simulink model "suspension"  (R2019a)
settings: Solver=ode15s  StartTime=0.0  StopTime=60  MaxStep=0.01  RelTol=1e-3  EnableMultiTasking=on
model workspace (MATLAB code in the model file):
  | dgrey = [0.3 0.3 0.3];
  | lgrey = [0.6 0.6 0.6];
  | orange = [255 140 0]/255;
  | blue = [0.0 0.6 0.8];
  | brown = [0.3 0.2 0.0];
  | lbrown = [167 108 52]/255;
  | yellow = [0.9 0.7 0.2];
  | red = [1.0 0.2 0.2];
  | black = [0 0 0];
  | 
  | rho_alum = 2700;
values from neighbouring files (symbols this model uses):
  back_frame_rad = intocm(0.25)    [loading.m]
  back_frame_thick_frame = intocm(0.25)    [loading.m]
  brake_disk_rad = intocm(3)    [loading.m]
  brake_disk_thick = intocm(0.25)    [loading.m]
  front_frame_rad = intocm(0.25)    [loading.m]
  front_frame_thick_frame = intocm(0.25)    [loading.m]
  hub_radius = intocm(2)    [loading.m]
  lower_left_link_len = intocm(link_upper)    [loading.m]
  lower_right_link_len = intocm(link_upper)    [loading.m]
  max_angle = 35    [loading.m]
  num_spokes = 4    [loading.m]
  outer_radius_spokes = intocm(5)    [loading.m]
  shaft_len = intocm(8)    [loading.m]
  shaft_rad = intocm(1.5)    [loading.m]
  steer_arm_chamfer = 0.25    [loading.m]
  steer_arm_height_forked = 13    [loading.m]
  steer_arm_len = 20    [loading.m]
  steer_arm_len_forked = 4    [loading.m]
  steer_arm_offset_forked = 3    [loading.m]
  steer_arm_pin_rad = 0.25    [loading.m]
  steer_arm_thick = 1    [loading.m]
  steer_arm_width = 2    [loading.m]
  steering_ball_rad = 1    [loading.m]
  steering_pin_height = 3    [loading.m]
  steering_pin_rad = 0.5    [loading.m]
  thickness_spokes = intocm(1)    [loading.m]
  tire_chamfer = 1    [loading.m]
  tire_density = 1000    [loading.m]
  tire_radius = intocm(9)    [loading.m]
  tire_width = intocm(7.5)    [loading.m]
  Ts = 60    [loading.m]
  upper_left_link_len = intocm(link_upper)    [loading.m]
  upper_right_link_len = intocm(link_upper)    [loading.m]
  upright_bearing_housing = 6    [loading.m]
  upright_chamfer = 0.3    [loading.m]
  upright_heigh_wheel = 8    [loading.m]
  upright_height = 43    [loading.m]
  upright_hub_thick = 2.5    [loading.m]
  upright_len = 8    [loading.m]
  upright_shaft_rad = 2.5    [loading.m]
  upright_thickness = 1    [loading.m]
  upright_trans_rad_to_wheel = 2    [loading.m]
  upright_width_wishbone = 10    [loading.m]
  width_hub = intocm(4.5)    [loading.m]
undefined symbols (not defined in the file or in its folder): sm_dwb_roadgen, X, Y, Z
libraries: sm_lib x75, sm_double_wishbone_suspension_lib x23, nesl_utility x18, simulink x3
(part 1 of 4)
Description:
  | Double Wishbone Suspension
  | 
  | This example illustrates a double wishbone front wheel automotive suspension. The suspension is
  | mounted on two platforms that can independently move up and down to simulate a road profile on
  | each wheel. For a given pair of road profiles, the resultant roll and bounce of the chassis can be
  | studied and the suspension parameters tuned for optimal performance. The inputs to the two
  | platforms are the road profile and its derivative. The platforms have a PD controller that controls
  | the vertical position of the platform to mimic the input road profile. See "Road Profiles Generator"
  | block dialog for details on the test road profiles.
  | 
  | Copyright 2008-2019 The MathWorks, Inc.
settings Model: Creator=MathWorks  LastModifiedBy=nicwiggins
settings DataIOCC: LimitDataPoints=on  SaveFormat=Array  SaveOutput=off  SaveTime=off  ReturnWorkspaceOutputs=off
settings OptimizationCC: ExpressionDepthLimit=2147483647  LifeSpan=inf
settings DebuggingCC: UnderspecifiedInitializationDetection=Classic  MergeDetectMultiDrivingBlocksExec=none  AllowSymbolicDim=off  StateNameClashWarn=warning  SFUnexpectedBacktrackingDiag=warning  SFNoUnconditionalDefaultTransitionDiag=warning  SFExecutionAtInitializationDiag=none  ArithmeticOperatorsInVariantConditions=warning
settings HardwareCC: ProdBitPerPointer=32  ProdBitPerSizeT=32  ProdBitPerPtrDiffT=32  ProdLargestAtomicFloat=None  ProdIntDivRoundTo=Undefined  ProdEndianess=Unspecified  ProdWordSize=32  ProdHWDeviceType=32-bit Generic
settings ModelReferenceCC: PropagateSignalLabelsOutOfModel=off
settings SFSimCC: SimUseLocalCustomCode=off  SimBuildMode=sf_make
settings RTWCC: RTWUseLocalCustomCode=off
settings CodeAppCC: StateflowObjectComments=on
settings GRTTargetCC: TargetLangStandard=C89/C90 (ANSI)  GeneratePreprocessorConditionals=Disable all
settings ConfigComp: CovMetricSettings=dw  CovHtmlReporting=on  CovSaveCumulativeToWorkspaceVar=on  CovSaveSingleToWorkspaceVar=on  CovExternalEMLEnable=off  CovSFcnEnable=off
settings SimscapeCC: SimscapeNormalizeSystem=off
settings ConfigurationSet: Description=SimMechanics 2G
settings DiagnosticsConfigSet: SimMechanicsUnconnectedFramePorts=none
settings ExplorerConfigSet: InternalSimMechanicsExplorerSettings="<ExplorerConfiguration><canonicalview>default</canonicalview><AnimationSetting><BasePlaybackSpeed>1.0</BasePlaybackSpeed><PlaybackSpeedFactor>1.0</PlaybackSpeedFactor></AnimationSetting><TilePanel><TileInfo><Tiles Columns=\"1\" Count=\"1\" Rows=\"1\"><Column Left=\"2\" Weight=\"1\"/><Column Left=\"827\"/><Row Top=\"2\" Weight=\"1\"/><Row Top=\"666\"/><Tile Height=\"1\" Width=\"1\" X=\"0\" Y=\"0\"/></Tiles></TileInfo><SceneInfo><SceneViewer><BGColor><R>0.60000002384185791</R><G>0.60000002384185791</G><B>0.60000002384185791</B></BGColor><Camera><Position><X>0</X><Y>-4.48140033882927202</Y><Z>0.554502487182617188</Z></Position><Center><X>0</X><Y>-0.245328903198242188</Y><Z>0.554502487182617188</Z></Center><Up><X>0</X><Y>-0</Y><Z>1</Z></Up><Left>-1.15500002503395094</Left><Right>1.15500002503395094</Right><Bottom>-0.792227599024772688</Bottom><Top>0.792227599024772688</Top></Camera></SceneViewer></SceneInfo></TilePanel></ExplorerConfiguration>"

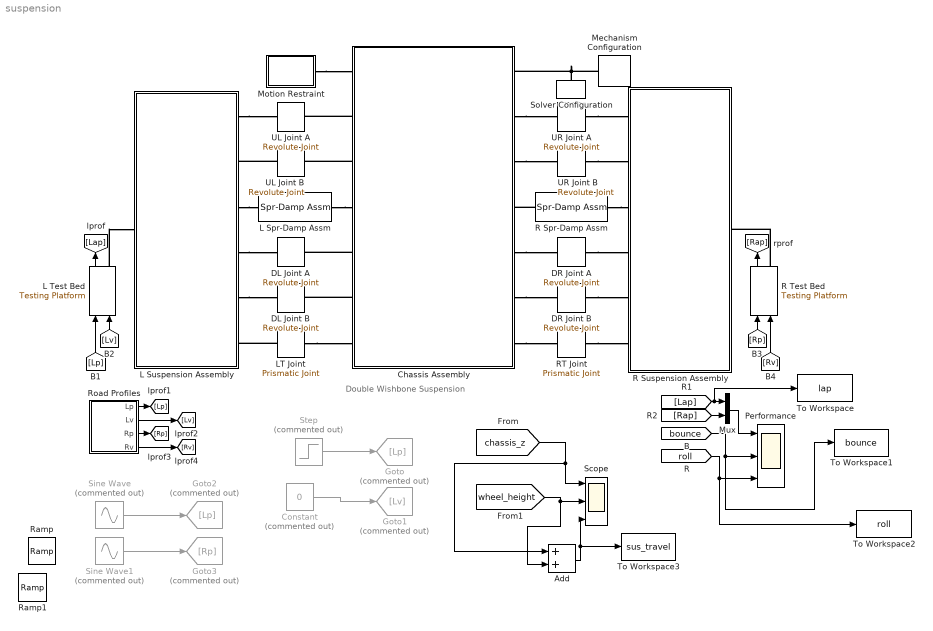
== system suspension ==
  note: Double Wishbone Suspension
  Add : Sum
  Chassis Assembly : Subsystem
      mask Display:
      | image(imread('sm_dwishbone_frameassm.png'));
      | port_label('LConn',1,'BC');
      | port_label('LConn',2,'ULA');
      | port_label('LConn',3,'ULB');
      | port_label('LConn',4,'ULC');
      | port_label('LConn',5,'DLA');
      | port_label('LConn',6,'DLB');
      | port_label('LConn',7,'LT');
      | port_label('RConn',1,'FC');
      | port_label('RConn',2,'URA');
      | port_label('RConn',3,'URB');
      | port_label('RConn',4,'URC');
      | port_label('RConn',5,'DRA');
      | port_label('RConn',6,'DRB');
      | port_label('RConn',7,'RT');
  Constant : Constant  Commented=on  Value=0
  DL Joint A : sm_lib/Joints/Revolute Joint  SenseConstraintForce=off  SenseConstraintForceX=off  SenseConstraintForceY=off  SenseConstraintForceZ=off  SenseConstraintTorque=off  SenseConstraintTorqueX=off  SenseConstraintTorqueY=off  SenseConstraintTorqueZ=off  SenseTotalForce=off  SenseTotalForceX=off  SenseTotalForceY=off  SenseTotalForceZ=off  SenseTotalTorque=off  SenseTotalTorqueX=off  SenseTotalTorqueY=off  SenseTotalTorqueZ=off  CompositeWrenchDir=FollowerOnBase  CompositeWrenchFrame=BaseFrame  EquilibriumPosition=0  EquilibriumPositionUnits=deg  SpringStiffness=0  SpringStiffnessUnits=N*m/deg  DampingCoefficient=0  DampingCoefficientUnits=N*m/(deg/s)  TorqueActuationMode=NoTorque  MotionActuationMode=ComputedMotion  SensePosition=off  SenseVelocity=off  SenseAcceleration=off  SenseTorqueForce=off  SenseLowerLimitTorqueForce=off  SenseUpperLimitTorqueForce=off  LowerLimitSpecify=off  LowerLimitBound=-90  LowerLimitBoundUnits=deg  LowerLimitStiffness=1e4  LowerLimitStiffnessUnits=N*m/deg  LowerLimitDamping=10  LowerLimitDampingUnits=N*m/(deg/s)  LowerLimitTransitionRegionWidth=0.1  LowerLimitTransitionRegionWidthUnits=deg  UpperLimitSpecify=off  UpperLimitBound=90  UpperLimitBoundUnits=deg  UpperLimitStiffness=1e4  UpperLimitStiffnessUnits=N*m/deg  UpperLimitDamping=10  UpperLimitDampingUnits=N*m/(deg/s)  UpperLimitTransitionRegionWidth=0.1  UpperLimitTransitionRegionWidthUnits=deg  PositionTargetSpecify=on  PositionTargetPriority=High  PositionTargetValue=0  PositionTargetValueUnits=deg  VelocityTargetSpecify=off  VelocityTargetPriority=High  VelocityTargetValue=0  VelocityTargetValueUnits=deg/s
  DL Joint B : sm_lib/Joints/Revolute Joint  SenseConstraintForce=off  SenseConstraintForceX=off  SenseConstraintForceY=off  SenseConstraintForceZ=off  SenseConstraintTorque=off  SenseConstraintTorqueX=off  SenseConstraintTorqueY=off  SenseConstraintTorqueZ=off  SenseTotalForce=off  SenseTotalForceX=off  SenseTotalForceY=off  SenseTotalForceZ=off  SenseTotalTorque=off  SenseTotalTorqueX=off  SenseTotalTorqueY=off  SenseTotalTorqueZ=off  CompositeWrenchDir=FollowerOnBase  CompositeWrenchFrame=BaseFrame  EquilibriumPosition=0  EquilibriumPositionUnits=deg  SpringStiffness=0  SpringStiffnessUnits=N*m/deg  DampingCoefficient=0  DampingCoefficientUnits=N*m/(deg/s)  TorqueActuationMode=NoTorque  MotionActuationMode=ComputedMotion  SensePosition=off  SenseVelocity=off  SenseAcceleration=off  SenseTorqueForce=off  SenseLowerLimitTorqueForce=off  SenseUpperLimitTorqueForce=off  LowerLimitSpecify=off  LowerLimitBound=-90  LowerLimitBoundUnits=deg  LowerLimitStiffness=1e4  LowerLimitStiffnessUnits=N*m/deg  LowerLimitDamping=10  LowerLimitDampingUnits=N*m/(deg/s)  LowerLimitTransitionRegionWidth=0.1  LowerLimitTransitionRegionWidthUnits=deg  UpperLimitSpecify=off  UpperLimitBound=90  UpperLimitBoundUnits=deg  UpperLimitStiffness=1e4  UpperLimitStiffnessUnits=N*m/deg  UpperLimitDamping=10  UpperLimitDampingUnits=N*m/(deg/s)  UpperLimitTransitionRegionWidth=0.1  UpperLimitTransitionRegionWidthUnits=deg  PositionTargetSpecify=off  PositionTargetPriority=High  PositionTargetValue=90  PositionTargetValueUnits=deg  VelocityTargetSpecify=off  VelocityTargetPriority=High  VelocityTargetValue=0  VelocityTargetValueUnits=deg/s
  DR Joint A : sm_lib/Joints/Revolute Joint  SenseConstraintForce=off  SenseConstraintForceX=off  SenseConstraintForceY=off  SenseConstraintForceZ=off  SenseConstraintTorque=off  SenseConstraintTorqueX=off  SenseConstraintTorqueY=off  SenseConstraintTorqueZ=off  SenseTotalForce=off  SenseTotalForceX=off  SenseTotalForceY=off  SenseTotalForceZ=off  SenseTotalTorque=off  SenseTotalTorqueX=off  SenseTotalTorqueY=off  SenseTotalTorqueZ=off  CompositeWrenchDir=FollowerOnBase  CompositeWrenchFrame=BaseFrame  EquilibriumPosition=0  EquilibriumPositionUnits=deg  SpringStiffness=0  SpringStiffnessUnits=N*m/deg  DampingCoefficient=0  DampingCoefficientUnits=N*m/(deg/s)  TorqueActuationMode=NoTorque  MotionActuationMode=ComputedMotion  SensePosition=off  SenseVelocity=off  SenseAcceleration=off  SenseTorqueForce=off  SenseLowerLimitTorqueForce=off  SenseUpperLimitTorqueForce=off  LowerLimitSpecify=off  LowerLimitBound=-90  LowerLimitBoundUnits=deg  LowerLimitStiffness=1e4  LowerLimitStiffnessUnits=N*m/deg  LowerLimitDamping=10  LowerLimitDampingUnits=N*m/(deg/s)  LowerLimitTransitionRegionWidth=0.1  LowerLimitTransitionRegionWidthUnits=deg  UpperLimitSpecify=off  UpperLimitBound=90  UpperLimitBoundUnits=deg  UpperLimitStiffness=1e4  UpperLimitStiffnessUnits=N*m/deg  UpperLimitDamping=10  UpperLimitDampingUnits=N*m/(deg/s)  UpperLimitTransitionRegionWidth=0.1  UpperLimitTransitionRegionWidthUnits=deg  PositionTargetSpecify=on  PositionTargetPriority=High  PositionTargetValue=0  PositionTargetValueUnits=deg  VelocityTargetSpecify=off  VelocityTargetPriority=High  VelocityTargetValue=0  VelocityTargetValueUnits=deg/s
  DR Joint B : sm_lib/Joints/Revolute Joint  SenseConstraintForce=off  SenseConstraintForceX=off  SenseConstraintForceY=off  SenseConstraintForceZ=off  SenseConstraintTorque=off  SenseConstraintTorqueX=off  SenseConstraintTorqueY=off  SenseConstraintTorqueZ=off  SenseTotalForce=off  SenseTotalForceX=off  SenseTotalForceY=off  SenseTotalForceZ=off  SenseTotalTorque=off  SenseTotalTorqueX=off  SenseTotalTorqueY=off  SenseTotalTorqueZ=off  CompositeWrenchDir=FollowerOnBase  CompositeWrenchFrame=BaseFrame  EquilibriumPosition=0  EquilibriumPositionUnits=deg  SpringStiffness=0  SpringStiffnessUnits=N*m/deg  DampingCoefficient=0  DampingCoefficientUnits=N*m/(deg/s)  TorqueActuationMode=NoTorque  MotionActuationMode=ComputedMotion  SensePosition=off  SenseVelocity=off  SenseAcceleration=off  SenseTorqueForce=off  SenseLowerLimitTorqueForce=off  SenseUpperLimitTorqueForce=off  LowerLimitSpecify=off  LowerLimitBound=-90  LowerLimitBoundUnits=deg  LowerLimitStiffness=1e4  LowerLimitStiffnessUnits=N*m/deg  LowerLimitDamping=10  LowerLimitDampingUnits=N*m/(deg/s)  LowerLimitTransitionRegionWidth=0.1  LowerLimitTransitionRegionWidthUnits=deg  UpperLimitSpecify=off  UpperLimitBound=90  UpperLimitBoundUnits=deg  UpperLimitStiffness=1e4  UpperLimitStiffnessUnits=N*m/deg  UpperLimitDamping=10  UpperLimitDampingUnits=N*m/(deg/s)  UpperLimitTransitionRegionWidth=0.1  UpperLimitTransitionRegionWidthUnits=deg  PositionTargetSpecify=off  PositionTargetPriority=High  PositionTargetValue=90  PositionTargetValueUnits=deg  VelocityTargetSpecify=off  VelocityTargetPriority=High  VelocityTargetValue=0  VelocityTargetValueUnits=deg/s
  Goto : Goto  Commented=on  GotoTag=Lp
  Goto1 : Goto  Commented=on  GotoTag=Lv
  Goto2 : Goto  Commented=on  GotoTag=Lp
  Goto3 : Goto  Commented=on  GotoTag=Rp
  L Test Bed : sm_double_wishbone_suspension_lib/Testing Platform  Ro=12  Ri=10  Rf=20  Tf=2  Hc=40  cclr=dgrey  loc=[-90 -25 0]  Rip=8  Hp=60  pclr=lgrey  L=40  W=40  H=3  clr=lgrey  Kp=1e4  Kd=100  rho=rho_alum
      settings: SourceProductName=Simscape Multibody  SourceProductBaseCode=MS
  L Spr-Damp Assm : sm_double_wishbone_suspension_lib/Spr-Damp Assm  Ks=100000  Kb=11000  Ls=18.5  Lc=22  Rci=2  Rco=3  Lp=16  Rr=0.3  Lb=6  Wb=4  Tb=1  Rbh=0.75  rho=rho_alum  cclr=yellow  pclr=brown
      settings: SourceProductName=Simscape Multibody  SourceProductBaseCode=MS
  L Suspension Assembly : Subsystem
      mask Display:
      | image(imread('sm_dwishbone_lwheelassm.png'));
      | 
      | port_label('LConn',1,'W');
      | 
      | port_label('RConn',1,'UA');
      | port_label('RConn',2,'UB');
      | port_label('RConn',3,'DP');
      | port_label('RConn',4,'DA');
      | port_label('RConn',5,'DB');
      | port_label('RConn',6,'LT');
  LT Joint : sm_lib/Joints/Prismatic Joint  SenseConstraintForce=off  SenseConstraintForceX=off  SenseConstraintForceY=off  SenseConstraintForceZ=off  SenseConstraintTorque=off  SenseConstraintTorqueX=off  SenseConstraintTorqueY=off  SenseConstraintTorqueZ=off  SenseTotalForce=off  SenseTotalForceX=off  SenseTotalForceY=off  SenseTotalForceZ=off  SenseTotalTorque=off  SenseTotalTorqueX=off  SenseTotalTorqueY=off  SenseTotalTorqueZ=off  CompositeWrenchDir=FollowerOnBase  CompositeWrenchFrame=BaseFrame  EquilibriumPosition=0  EquilibriumPositionUnits=m  SpringStiffness=0  SpringStiffnessUnits=N/m  DampingCoefficient=0  DampingCoefficientUnits=N/(m/s)  TorqueActuationMode=NoTorque  MotionActuationMode=ComputedMotion  SensePosition=off  SenseVelocity=off  SenseAcceleration=off  SenseTorqueForce=off  SenseLowerLimitTorqueForce=off  SenseUpperLimitTorqueForce=off  LowerLimitSpecify=off  LowerLimitBound=-1  LowerLimitBoundUnits=m  LowerLimitStiffness=1e6  LowerLimitStiffnessUnits=N/m  LowerLimitDamping=1e3  LowerLimitDampingUnits=N/(m/s)  LowerLimitTransitionRegionWidth=1e-4  LowerLimitTransitionRegionWidthUnits=m  UpperLimitSpecify=off  UpperLimitBound=1  UpperLimitBoundUnits=m  UpperLimitStiffness=1e6  UpperLimitStiffnessUnits=N/m  UpperLimitDamping=1e3  UpperLimitDampingUnits=N/(m/s)  UpperLimitTransitionRegionWidth=1e-4  UpperLimitTransitionRegionWidthUnits=m  PositionTargetSpecify=off  PositionTargetPriority=High  PositionTargetValue=0  PositionTargetValueUnits=m  VelocityTargetSpecify=off  VelocityTargetPriority=High  VelocityTargetValue=0  VelocityTargetValueUnits=m/s
  Mechanism Configuration : sm_lib/Utilities/Mechanism Configuration  UniformGravity=Constant  GravityVector=[0 0 -9.81]  GravityUnits=m/s^2  LinearizationDelta=0.001
  Motion Restraint : Subsystem
  Mux : Mux  Inputs=2
  Performance : Scope  NumInputPorts=3
  R Test Bed : sm_double_wishbone_suspension_lib/Testing Platform  Ro=12  Ri=10  Rf=20  Tf=2  Hc=40  cclr=dgrey  loc=[90 -25 0]  Rip=8  Hp=60  pclr=lgrey  L=40  W=40  H=3  clr=lgrey  Kp=1e4  Kd=100  rho=rho_alum
      settings: SourceProductName=Simscape Multibody  SourceProductBaseCode=MS
  R Spr-Damp Assm : sm_double_wishbone_suspension_lib/Spr-Damp Assm  Ks=100000  Kb=11000  Ls=18.5  Lc=22  Rci=2  Rco=3  Lp=16  Rr=0.3  Lb=6  Wb=4  Tb=1  Rbh=0.75  rho=rho_alum  cclr=yellow  pclr=brown
      settings: SourceProductName=Simscape Multibody  SourceProductBaseCode=MS
  R Suspension Assembly : Subsystem
      mask Display:
      | image(imread('sm_dwishbone_rwheelassm.png'));
      | 
      | port_label('RConn',1,'T');
      | 
      | port_label('LConn',1,'UA');
      | port_label('LConn',2,'UB');
      | port_label('LConn',3,'DP');
      | port_label('LConn',4,'DA');
      | port_label('LConn',5,'DB');
      | port_label('LConn',6,'RT');
  RT Joint : sm_lib/Joints/Prismatic Joint  SenseConstraintForce=off  SenseConstraintForceX=off  SenseConstraintForceY=off  SenseConstraintForceZ=off  SenseConstraintTorque=off  SenseConstraintTorqueX=off  SenseConstraintTorqueY=off  SenseConstraintTorqueZ=off  SenseTotalForce=off  SenseTotalForceX=off  SenseTotalForceY=off  SenseTotalForceZ=off  SenseTotalTorque=off  SenseTotalTorqueX=off  SenseTotalTorqueY=off  SenseTotalTorqueZ=off  CompositeWrenchDir=FollowerOnBase  CompositeWrenchFrame=BaseFrame  EquilibriumPosition=0  EquilibriumPositionUnits=m  SpringStiffness=0  SpringStiffnessUnits=N/m  DampingCoefficient=0  DampingCoefficientUnits=N/(m/s)  TorqueActuationMode=NoTorque  MotionActuationMode=ComputedMotion  SensePosition=off  SenseVelocity=off  SenseAcceleration=off  SenseTorqueForce=off  SenseLowerLimitTorqueForce=off  SenseUpperLimitTorqueForce=off  LowerLimitSpecify=off  LowerLimitBound=-1  LowerLimitBoundUnits=m  LowerLimitStiffness=1e6  LowerLimitStiffnessUnits=N/m  LowerLimitDamping=1e3  LowerLimitDampingUnits=N/(m/s)  LowerLimitTransitionRegionWidth=1e-4  LowerLimitTransitionRegionWidthUnits=m  UpperLimitSpecify=off  UpperLimitBound=1  UpperLimitBoundUnits=m  UpperLimitStiffness=1e6  UpperLimitStiffnessUnits=N/m  UpperLimitDamping=1e3  UpperLimitDampingUnits=N/(m/s)  UpperLimitTransitionRegionWidth=1e-4  UpperLimitTransitionRegionWidthUnits=m  PositionTargetSpecify=off  PositionTargetPriority=High  PositionTargetValue=0  PositionTargetValueUnits=m  VelocityTargetSpecify=off  VelocityTargetPriority=High  VelocityTargetValue=0  VelocityTargetValueUnits=m/s
  Ramp : simulink/Sources/Ramp  slope=1  start=0  InitialOutput=-10
  Ramp1 : simulink/Sources/Ramp  slope=1  start=0  InitialOutput=10
  Road Profiles : Subsystem  mask(Road Profile Generator){Ti=2, Ts=5.5, Tb=1, Fl=0.5, Al=5, Fm=3, Am=5, Fh=5, Ah=5, Ps=2, As=5, Wp=0.1, Pp=2, Ap=5, Ad=25}
      mask prompts: Ti "Start time (s):"; Ts "Duration of each segment (s):"; Tb "Buffer between segments (s):"; Fl "Frequency (Hz):"; Al "Amplitude (cm):"; Fm "Frequency (Hz):"; Am "Amplitude (cm):"; Fh "Frequency (Hz):"; Ah "Amplitude (cm):"; Ps "Period (s):"; As "Amplitude (cm):"; Wp "Width (s):"; Pp "Period (s):"; Ap "Amplitude (cm):"; Ad "Depth (cm):"
      mask help:
      | This block generates test road profiles for the left and right tires. A road profile is comprised of the following
      | 1  - Low frequency sinusoid with the left and right road profiles in phase
      | 2  - Low frequency sinusoid with the left and right road profiles out of phase
      | 3  - Mid frequency sinusoid with the left and right road profiles in phase
      | 4  - Mid frequency sinusoid with the left and right road profiles out of phase
      | 5  - High frequency sinusoid with the left and right road profiles in phase
      | 6  - High frequency sinusoid with the left and right road profiles out of phase
      | 7  - Step with the left and right road profiles in phase
      | 8  - Step with the left and right road profiles out of phase
      | 9  - Pulse with the left and right road profiles in phase
      | 10 - Pulse with the left and right road profiles out of phase
      | 11 - Large step down (Dive)
      mask Display:
      | image(imread('sm_dwishbone_road.png'));
      | port_label('output',1,'Lp');
      | port_label('output',2,'Lv');
      | port_label('output',3,'Rp');
      | port_label('output',4,'Rv');
  Scope : Scope  NumInputPorts=3
  Sine Wave : Sin  Commented=on  Amplitude=10  Frequency=3  SampleTime=0
  Sine Wave1 : Sin  Commented=on  Amplitude=10  Frequency=3  SampleTime=0
  Solver Configuration : nesl_utility/Solver Configuration  PhysicalDomain=network_engine_domain  SubClassName=solver  LeftPortType=input  RightPortType=generic  Tones=[]  Harmonics=[]  SimulateNoise=off  Profile=off  UseLocalSampling=off  EnableSwitchedLinearOptims=on  FrequencyDomain=off  UseCCode=off  RelTol=0.001  AbsTol=1e-06  MinStep=1e-09  ToWorkspace=off  RevertToSquareIcSolve=off  NumHomotopyIterations=100  PhasorMode=off  PhasorModeNumHarmonics=1  DoDC=off  ResidualTolerance=1e-6  UseLocalSolver=off  LocalSolverChoice=NE_BACKWARD_EULER_ADVANCER  LocalSolverSampleTime=.001  DoFixedCost=off  MaxNonlinIter=3  MaxModeIter=2  LinearAlgebra=Sparse  EquationFormulation=NE_TIME_EF  DelaysMemoryBudget=1024  AutomaticFiltering=on  FilteringTimeConstant=0.001  PartitionStorageMethod=AS_NEEDED  PartitionMemoryBudget=1024  PartitionMethod=FAST
  Step : Step  Commented=on  SampleTime=0
  To Workspace : ToWorkspace  VariableName=lap  SaveFormat=Timeseries  SampleTime=-1
  To Workspace1 : ToWorkspace  VariableName=bounce  SaveFormat=Timeseries  SampleTime=-1
  To Workspace2 : ToWorkspace  VariableName=roll  SaveFormat=Timeseries  SampleTime=-1
  To Workspace3 : ToWorkspace  VariableName=sus_travel  SaveFormat=Timeseries  SampleTime=-1
  UL Joint A : sm_lib/Joints/Revolute Joint  SenseConstraintForce=off  SenseConstraintForceX=off  SenseConstraintForceY=off  SenseConstraintForceZ=off  SenseConstraintTorque=off  SenseConstraintTorqueX=off  SenseConstraintTorqueY=off  SenseConstraintTorqueZ=off  SenseTotalForce=off  SenseTotalForceX=off  SenseTotalForceY=off  SenseTotalForceZ=off  SenseTotalTorque=off  SenseTotalTorqueX=off  SenseTotalTorqueY=off  SenseTotalTorqueZ=off  CompositeWrenchDir=FollowerOnBase  CompositeWrenchFrame=BaseFrame  EquilibriumPosition=0  EquilibriumPositionUnits=deg  SpringStiffness=0  SpringStiffnessUnits=N*m/deg  DampingCoefficient=0  DampingCoefficientUnits=N*m/(deg/s)  TorqueActuationMode=NoTorque  MotionActuationMode=ComputedMotion  SensePosition=off  SenseVelocity=off  SenseAcceleration=off  SenseTorqueForce=off  SenseLowerLimitTorqueForce=off  SenseUpperLimitTorqueForce=off  LowerLimitSpecify=off  LowerLimitBound=-90  LowerLimitBoundUnits=deg  LowerLimitStiffness=1e4  LowerLimitStiffnessUnits=N*m/deg  LowerLimitDamping=10  LowerLimitDampingUnits=N*m/(deg/s)  LowerLimitTransitionRegionWidth=0.1  LowerLimitTransitionRegionWidthUnits=deg  UpperLimitSpecify=off  UpperLimitBound=90  UpperLimitBoundUnits=deg  UpperLimitStiffness=1e4  UpperLimitStiffnessUnits=N*m/deg  UpperLimitDamping=10  UpperLimitDampingUnits=N*m/(deg/s)  UpperLimitTransitionRegionWidth=0.1  UpperLimitTransitionRegionWidthUnits=deg  PositionTargetSpecify=off  PositionTargetPriority=Low  PositionTargetValue=180  PositionTargetValueUnits=deg  VelocityTargetSpecify=off  VelocityTargetPriority=High  VelocityTargetValue=0  VelocityTargetValueUnits=deg/s
  UL Joint B : sm_lib/Joints/Revolute Joint  SenseConstraintForce=off  SenseConstraintForceX=off  SenseConstraintForceY=off  SenseConstraintForceZ=off  SenseConstraintTorque=off  SenseConstraintTorqueX=off  SenseConstraintTorqueY=off  SenseConstraintTorqueZ=off  SenseTotalForce=off  SenseTotalForceX=off  SenseTotalForceY=off  SenseTotalForceZ=off  SenseTotalTorque=off  SenseTotalTorqueX=off  SenseTotalTorqueY=off  SenseTotalTorqueZ=off  CompositeWrenchDir=FollowerOnBase  CompositeWrenchFrame=BaseFrame  EquilibriumPosition=0  EquilibriumPositionUnits=deg  SpringStiffness=0  SpringStiffnessUnits=N*m/deg  DampingCoefficient=0  DampingCoefficientUnits=N*m/(deg/s)  TorqueActuationMode=NoTorque  MotionActuationMode=ComputedMotion  SensePosition=off  SenseVelocity=off  SenseAcceleration=off  SenseTorqueForce=off  SenseLowerLimitTorqueForce=off  SenseUpperLimitTorqueForce=off  LowerLimitSpecify=off  LowerLimitBound=-90  LowerLimitBoundUnits=deg  LowerLimitStiffness=1e4  LowerLimitStiffnessUnits=N*m/deg  LowerLimitDamping=10  LowerLimitDampingUnits=N*m/(deg/s)  LowerLimitTransitionRegionWidth=0.1  LowerLimitTransitionRegionWidthUnits=deg  UpperLimitSpecify=off  UpperLimitBound=90  UpperLimitBoundUnits=deg  UpperLimitStiffness=1e4  UpperLimitStiffnessUnits=N*m/deg  UpperLimitDamping=10  UpperLimitDampingUnits=N*m/(deg/s)  UpperLimitTransitionRegionWidth=0.1  UpperLimitTransitionRegionWidthUnits=deg  PositionTargetSpecify=off  PositionTargetPriority=High  PositionTargetValue=90  PositionTargetValueUnits=deg  VelocityTargetSpecify=off  VelocityTargetPriority=High  VelocityTargetValue=0  VelocityTargetValueUnits=deg/s
  UR Joint A : sm_lib/Joints/Revolute Joint  SenseConstraintForce=off  SenseConstraintForceX=off  SenseConstraintForceY=off  SenseConstraintForceZ=off  SenseConstraintTorque=off  SenseConstraintTorqueX=off  SenseConstraintTorqueY=off  SenseConstraintTorqueZ=off  SenseTotalForce=off  SenseTotalForceX=off  SenseTotalForceY=off  SenseTotalForceZ=off  SenseTotalTorque=off  SenseTotalTorqueX=off  SenseTotalTorqueY=off  SenseTotalTorqueZ=off  CompositeWrenchDir=FollowerOnBase  CompositeWrenchFrame=BaseFrame  EquilibriumPosition=0  EquilibriumPositionUnits=deg  SpringStiffness=0  SpringStiffnessUnits=N*m/deg  DampingCoefficient=0  DampingCoefficientUnits=N*m/(deg/s)  TorqueActuationMode=NoTorque  MotionActuationMode=ComputedMotion  SensePosition=off  SenseVelocity=off  SenseAcceleration=off  SenseTorqueForce=off  SenseLowerLimitTorqueForce=off  SenseUpperLimitTorqueForce=off  LowerLimitSpecify=off  LowerLimitBound=-90  LowerLimitBoundUnits=deg  LowerLimitStiffness=1e4  LowerLimitStiffnessUnits=N*m/deg  LowerLimitDamping=10  LowerLimitDampingUnits=N*m/(deg/s)  LowerLimitTransitionRegionWidth=0.1  LowerLimitTransitionRegionWidthUnits=deg  UpperLimitSpecify=off  UpperLimitBound=90  UpperLimitBoundUnits=deg  UpperLimitStiffness=1e4  UpperLimitStiffnessUnits=N*m/deg  UpperLimitDamping=10  UpperLimitDampingUnits=N*m/(deg/s)  UpperLimitTransitionRegionWidth=0.1  UpperLimitTransitionRegionWidthUnits=deg  PositionTargetSpecify=off  PositionTargetPriority=High  PositionTargetValue=90  PositionTargetValueUnits=deg  VelocityTargetSpecify=off  VelocityTargetPriority=High  VelocityTargetValue=0  VelocityTargetValueUnits=deg/s
  UR Joint B : sm_lib/Joints/Revolute Joint  SenseConstraintForce=off  SenseConstraintForceX=off  SenseConstraintForceY=off  SenseConstraintForceZ=off  SenseConstraintTorque=off  SenseConstraintTorqueX=off  SenseConstraintTorqueY=off  SenseConstraintTorqueZ=off  SenseTotalForce=off  SenseTotalForceX=off  SenseTotalForceY=off  SenseTotalForceZ=off  SenseTotalTorque=off  SenseTotalTorqueX=off  SenseTotalTorqueY=off  SenseTotalTorqueZ=off  CompositeWrenchDir=FollowerOnBase  CompositeWrenchFrame=BaseFrame  EquilibriumPosition=0  EquilibriumPositionUnits=deg  SpringStiffness=0  SpringStiffnessUnits=N*m/deg  DampingCoefficient=0  DampingCoefficientUnits=N*m/(deg/s)  TorqueActuationMode=NoTorque  MotionActuationMode=ComputedMotion  SensePosition=off  SenseVelocity=off  SenseAcceleration=off  SenseTorqueForce=off  SenseLowerLimitTorqueForce=off  SenseUpperLimitTorqueForce=off  LowerLimitSpecify=off  LowerLimitBound=-90  LowerLimitBoundUnits=deg  LowerLimitStiffness=1e4  LowerLimitStiffnessUnits=N*m/deg  LowerLimitDamping=10  LowerLimitDampingUnits=N*m/(deg/s)  LowerLimitTransitionRegionWidth=0.1  LowerLimitTransitionRegionWidthUnits=deg  UpperLimitSpecify=off  UpperLimitBound=90  UpperLimitBoundUnits=deg  UpperLimitStiffness=1e4  UpperLimitStiffnessUnits=N*m/deg  UpperLimitDamping=10  UpperLimitDampingUnits=N*m/(deg/s)  UpperLimitTransitionRegionWidth=0.1  UpperLimitTransitionRegionWidthUnits=deg  PositionTargetSpecify=off  PositionTargetPriority=High  PositionTargetValue=0  PositionTargetValueUnits=deg  VelocityTargetSpecify=off  VelocityTargetPriority=High  VelocityTargetValue=0  VelocityTargetValueUnits=deg/s
  wires:
  [bounce] -> To Workspace1/1, Performance/2
  [roll] -> To Workspace2/1, Performance/3
  [Lap] -> To Workspace/1, Mux/1
  [Rap] -> Mux/2
  Mux/1 -> Performance/1
  R Test Bed/1 -> [Rap]
  Road Profiles/1(Lp) -> [Lp]
  Road Profiles/2(Lv) -> [Lv]
  Road Profiles/3(Rp) -> [Rp]
  Road Profiles/4(Rv) -> [Rv]
  [Rp] -> R Test Bed/1
  [Rv] -> R Test Bed/2
  [Lp] -> L Test Bed/1
  [Lv] -> L Test Bed/2
  L Test Bed/1 -> [Lap]
  Step/1 -> Goto/1
  Constant/1 -> Goto1/1
  [wheel_height] -> Add/2, Scope/2
  [chassis_z] -> Add/1, Scope/1
  Add/1 -> Scope/3, To Workspace3/1
  Sine Wave/1 -> Goto2/1
  Sine Wave1/1 -> Goto3/1
  connections:
  UR Joint A/RConn1 -- R Suspension Assembly/LConn1
  UR Joint B/RConn1 -- R Suspension Assembly/LConn2
  DR Joint A/RConn1 -- R Suspension Assembly/LConn4
  DR Joint B/RConn1 -- R Suspension Assembly/LConn5
  Chassis Assembly/RConn2 -- UR Joint A/LConn1
  Chassis Assembly/RConn3 -- UR Joint B/LConn1
  Chassis Assembly/RConn5 -- DR Joint A/LConn1
  Chassis Assembly/RConn6 -- DR Joint B/LConn1
  R Spr-Damp Assm/LConn1 -- Chassis Assembly/RConn4
  R Spr-Damp Assm/RConn1 -- R Suspension Assembly/LConn3
  R Test Bed/RConn1 -- R Suspension Assembly/RConn1
  Mechanism Configuration/RConn1 -- Solver Configuration/RConn1 -- Chassis Assembly/RConn1
  Motion Restraint/RConn1 -- Chassis Assembly/LConn1
  Chassis Assembly/LConn6 -- DL Joint B/LConn1
  UL Joint B/RConn1 -- L Suspension Assembly/RConn2
  Chassis Assembly/LConn3 -- UL Joint B/LConn1
  L Suspension Assembly/RConn1 -- UL Joint A/RConn1
  L Suspension Assembly/RConn5 -- DL Joint B/RConn1
  L Suspension Assembly/RConn4 -- DL Joint A/RConn1
  Chassis Assembly/LConn5 -- DL Joint A/LConn1
  Chassis Assembly/LConn2 -- UL Joint A/LConn1
  L Spr-Damp Assm/LConn1 -- Chassis Assembly/LConn4
  Chassis Assembly/RConn7 -- RT Joint/LConn1
  L Suspension Assembly/RConn3 -- L Spr-Damp Assm/RConn1
  RT Joint/RConn1 -- R Suspension Assembly/LConn6
  LT Joint/LConn1 -- Chassis Assembly/LConn7
  LT Joint/RConn1 -- L Suspension Assembly/RConn6
  L Test Bed/RConn1 -- L Suspension Assembly/LConn1

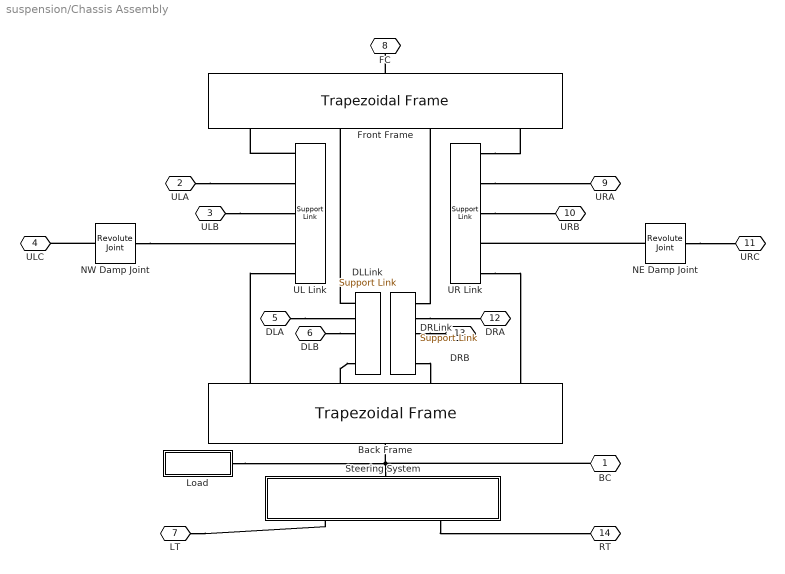
== system suspension/Chassis Assembly ==
  Back Frame : sm_double_wishbone_suspension_lib/Trapezoidal Frame  L1=back_frame_up  L2=back_frame_low  H=back_frame_height  R=back_frame_rad  T=back_frame_thick_frame  Tb=back_frame_thick_frame_bar  rho=rho_alum  clr=orange
      settings: SourceProductName=Simscape Multibody  SourceProductBaseCode=MS
  DLLink : sm_double_wishbone_suspension_lib/Support Link  L=lower_left_link_len  Ro=1.5  Ri=0.75  Lw=5.5  Ls=1  Ld=10.25  Ow=5.125  Rr=0.2  rho=rho_alum  clr=orange
      settings: SourceProductName=Simscape Multibody  SourceProductBaseCode=MS
  DRLink : sm_double_wishbone_suspension_lib/Support Link  L=lower_right_link_len  Ro=1.5  Ri=0.75  Lw=5.5  Ls=1  Ld=10.25  Ow=5.125  Rr=0.2  rho=rho_alum  clr=orange
      settings: SourceProductName=Simscape Multibody  SourceProductBaseCode=MS
  Front Frame : sm_double_wishbone_suspension_lib/Trapezoidal Frame  L1=front_frame_up  L2=front_frame_low  H=front_frame_height  R=front_frame_rad  T=front_frame_thick_frame  Tb=front_frame_thick_frame_bar  rho=rho_alum  clr=orange
      settings: SourceProductName=Simscape Multibody  SourceProductBaseCode=MS
  Load : Subsystem
  NE Damp Joint : sm_lib/Joints/Revolute Joint  SenseConstraintForce=off  SenseConstraintForceX=off  SenseConstraintForceY=off  SenseConstraintForceZ=off  SenseConstraintTorque=off  SenseConstraintTorqueX=off  SenseConstraintTorqueY=off  SenseConstraintTorqueZ=off  SenseTotalForce=off  SenseTotalForceX=off  SenseTotalForceY=off  SenseTotalForceZ=off  SenseTotalTorque=off  SenseTotalTorqueX=off  SenseTotalTorqueY=off  SenseTotalTorqueZ=off  CompositeWrenchDir=FollowerOnBase  CompositeWrenchFrame=BaseFrame  EquilibriumPosition=0  EquilibriumPositionUnits=deg  SpringStiffness=0  SpringStiffnessUnits=N*m/deg  DampingCoefficient=0  DampingCoefficientUnits=N*m/(deg/s)  TorqueActuationMode=NoTorque  MotionActuationMode=ComputedMotion  SensePosition=off  SenseVelocity=off  SenseAcceleration=off  SenseTorqueForce=off  SenseLowerLimitTorqueForce=off  SenseUpperLimitTorqueForce=off  LowerLimitSpecify=off  LowerLimitBound=-90  LowerLimitBoundUnits=deg  LowerLimitStiffness=1e4  LowerLimitStiffnessUnits=N*m/deg  LowerLimitDamping=10  LowerLimitDampingUnits=N*m/(deg/s)  LowerLimitTransitionRegionWidth=0.1  LowerLimitTransitionRegionWidthUnits=deg  UpperLimitSpecify=off  UpperLimitBound=90  UpperLimitBoundUnits=deg  UpperLimitStiffness=1e4  UpperLimitStiffnessUnits=N*m/deg  UpperLimitDamping=10  UpperLimitDampingUnits=N*m/(deg/s)  UpperLimitTransitionRegionWidth=0.1  UpperLimitTransitionRegionWidthUnits=deg  PositionTargetSpecify=off  PositionTargetPriority=High  PositionTargetValue=0  PositionTargetValueUnits=deg  VelocityTargetSpecify=off  VelocityTargetPriority=High  VelocityTargetValue=0  VelocityTargetValueUnits=deg/s
  NW Damp Joint : sm_lib/Joints/Revolute Joint  SenseConstraintForce=off  SenseConstraintForceX=off  SenseConstraintForceY=off  SenseConstraintForceZ=off  SenseConstraintTorque=off  SenseConstraintTorqueX=off  SenseConstraintTorqueY=off  SenseConstraintTorqueZ=off  SenseTotalForce=off  SenseTotalForceX=off  SenseTotalForceY=off  SenseTotalForceZ=off  SenseTotalTorque=off  SenseTotalTorqueX=off  SenseTotalTorqueY=off  SenseTotalTorqueZ=off  CompositeWrenchDir=FollowerOnBase  CompositeWrenchFrame=BaseFrame  EquilibriumPosition=0  EquilibriumPositionUnits=deg  SpringStiffness=0  SpringStiffnessUnits=N*m/deg  DampingCoefficient=0  DampingCoefficientUnits=N*m/(deg/s)  TorqueActuationMode=NoTorque  MotionActuationMode=ComputedMotion  SensePosition=off  SenseVelocity=off  SenseAcceleration=off  SenseTorqueForce=off  SenseLowerLimitTorqueForce=off  SenseUpperLimitTorqueForce=off  LowerLimitSpecify=off  LowerLimitBound=-90  LowerLimitBoundUnits=deg  LowerLimitStiffness=1e4  LowerLimitStiffnessUnits=N*m/deg  LowerLimitDamping=10  LowerLimitDampingUnits=N*m/(deg/s)  LowerLimitTransitionRegionWidth=0.1  LowerLimitTransitionRegionWidthUnits=deg  UpperLimitSpecify=off  UpperLimitBound=90  UpperLimitBoundUnits=deg  UpperLimitStiffness=1e4  UpperLimitStiffnessUnits=N*m/deg  UpperLimitDamping=10  UpperLimitDampingUnits=N*m/(deg/s)  UpperLimitTransitionRegionWidth=0.1  UpperLimitTransitionRegionWidthUnits=deg  PositionTargetSpecify=off  PositionTargetPriority=High  PositionTargetValue=0  PositionTargetValueUnits=deg  VelocityTargetSpecify=off  VelocityTargetPriority=High  VelocityTargetValue=0  VelocityTargetValueUnits=deg/s
  Steering System : Subsystem
      mask Display:
      | image(imread('sm_dwishbone_steeringsys.png'));
      | port_label('LConn',1,'B');
      | port_label('RConn',1,'LT');
      | port_label('RConn',2,'RT');
  UL Link : sm_double_wishbone_suspension_lib/Support Link  L=upper_left_link_len  Ro=1.5  Ri=0.75  Lw=5.5  Ls=3  Ld=20.5  Ow=0  Rr=0.2  rho=rho_alum  clr=orange
      settings: SourceProductName=Simscape Multibody  SourceProductBaseCode=MS
  UR Link : sm_double_wishbone_suspension_lib/Support Link  L=upper_right_link_len  Ro=1.5  Ri=0.75  Lw=5.5  Ls=3  Ld=20.5  Ow=0  Rr=0.2  rho=rho_alum  clr=orange
      settings: SourceProductName=Simscape Multibody  SourceProductBaseCode=MS
  BC : PMIOPort  Side=Left
  ULA : PMIOPort  Port=2  Side=Left
  ULB : PMIOPort  Port=3  Side=Left
  ULC : PMIOPort  Port=4  Side=Left
  DLA : PMIOPort  Port=5  Side=Left
  DLB : PMIOPort  Port=6  Side=Left
  LT : PMIOPort  Port=7  Side=Left
  FC : PMIOPort  Port=8  Side=Right
  URA : PMIOPort  Port=9  Side=Right
  URB : PMIOPort  Port=10  Side=Right
  URC : PMIOPort  Port=11  Side=Right
  DRA : PMIOPort  Port=12  Side=Right
  DRB : PMIOPort  Port=13  Side=Right
  RT : PMIOPort  Port=14  Side=Right
  connections:
  DRLink/LConn3 -- DRB/RConn1
  DRLink/LConn2 -- DRA/RConn1
  DLA/RConn1 -- DLLink/LConn2
  DLB/RConn1 -- DLLink/LConn3
  UR Link/LConn3 -- URB/RConn1
  UR Link/LConn2 -- URA/RConn1
  DLLink/LConn1 -- Front Frame/LConn2
  UR Link/LConn1 -- Front Frame/LConn4
  Back Frame/LConn2 -- DLLink/LConn5
  DRLink/LConn1 -- Front Frame/LConn3
  ULB/RConn1 -- UL Link/LConn3
  DRLink/LConn5 -- Back Frame/LConn3
  Front Frame/RConn1 -- FC/RConn1
  UR Link/LConn5 -- Back Frame/LConn4
  Back Frame/LConn1 -- UL Link/LConn5
  ULA/RConn1 -- UL Link/LConn2
  UL Link/LConn1 -- Front Frame/LConn1
  Steering System/LConn1 -- Back Frame/RConn1 -- Load/RConn1 -- BC/RConn1
  LT/RConn1 -- Steering System/RConn1
  Steering System/RConn2 -- RT/RConn1
  NW Damp Joint/LConn1 -- UL Link/LConn4
  NW Damp Joint/RConn1 -- ULC/RConn1
  NE Damp Joint/LConn1 -- UR Link/LConn4
  NE Damp Joint/RConn1 -- URC/RConn1
